simulink model "UnitTest_2"  (R2018b)
settings: Solver=FixedStepAuto  StartTime=0.0  StopTime=tfinal  FixedStep=1/30  RelTol=1e-3
values from neighbouring files (symbols this model uses):
  Bb = [14491; 3674; 39514] *1e-9    [UnitTestScript.m]
  Ri = [0.1;1;0.025]    [UnitTestScript.m]
libraries: aerolibutil x2, MEKF_lib x1
settings Model: Creator=kylle  LastModifiedBy=kylle

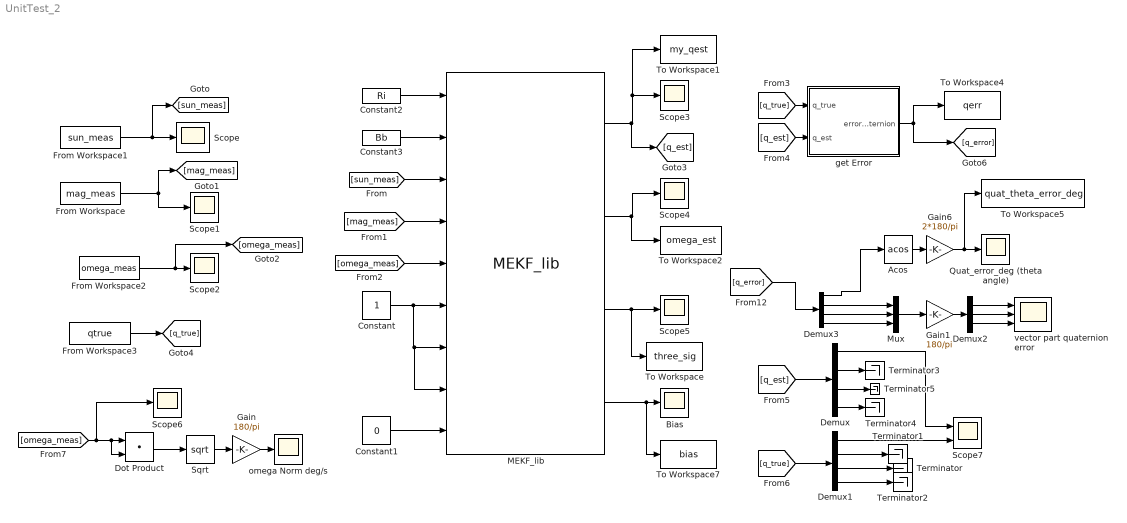
== system UnitTest_2 ==
  Acos : Trigonometry  Operator=acos
  Bias : Scope
  Constant : Constant
  Constant1 : Constant  Value=0
  Constant2 : Constant  Value=Ri
  Constant3 : Constant  Value=Bb
  Demux : Demux
  Demux1 : Demux
  Demux2 : Demux  Outputs=3
  Demux3 : Demux
  Dot Product : DotProduct  InputSameDT=on  OutDataTypeStr=Inherit: Inherit via internal rule
  From Workspace : FromWorkspace  VariableName=mag_meas  SampleTime=0
  From Workspace1 : FromWorkspace  VariableName=sun_meas  SampleTime=0
  From Workspace2 : FromWorkspace  VariableName=omega_meas  SampleTime=0
  From Workspace3 : FromWorkspace  VariableName=qtrue  SampleTime=0
  Gain : Gain  Gain=180/pi
  Gain1 : Gain  Gain=180/pi
  Gain6 : Gain  Gain=2*180/pi
  MEKF_lib : MEKF_lib/MEKF_lib  SystemSampleTime=-1
  Mux : Mux  Inputs=3
  Quat_error_deg (theta angle) : Scope
  Scope{,1..6} (7 alike) : Scope
  Scope7 : Scope  NumInputPorts=2
  Sqrt : Sqrt  SaturateOnIntegerOverflow=on
  Terminator{,1..5} (6 alike) : Terminator
  To Workspace : ToWorkspace  VariableName=three_sig  SaveFormat=Structure With Time  SampleTime=-1
  To Workspace1 : ToWorkspace  VariableName=my_qest  SaveFormat=Structure With Time  SampleTime=-1
  To Workspace2 : ToWorkspace  VariableName=omega_est  SaveFormat=Structure  SampleTime=-1
  To Workspace4 : ToWorkspace  VariableName=qerr  SaveFormat=Structure With Time  SampleTime=-1
  To Workspace5 : ToWorkspace  VariableName=quat_theta_error_deg  SaveFormat=Structure With Time  SampleTime=-1
  To Workspace7 : ToWorkspace  VariableName=bias  SaveFormat=Structure With Time  SampleTime=-1
  get Error : Subsystem
  omega Norm deg/s : Scope
  vector part quaternion error : Scope  NumInputPorts=3
  wires:
  Constant/1 -> MEKF_lib/8, MEKF_lib/7, MEKF_lib/6
  From Workspace1/1 -> [sun_meas], Scope/1
  From Workspace/1 -> [mag_meas], Scope1/1
  From Workspace2/1 -> [omega_meas], Scope2/1
  get Error/1(error_quaternion) -> To Workspace4/1, [q_error]
  [q_est] -> get Error/2(q_est)
  [q_true] -> get Error/1(q_true)
  From Workspace3/1 -> [q_true]
  Gain6/1 -> To Workspace5/1, Quat_error_deg (theta angle)/1
  Demux3/1 -> Acos/1
  Acos/1 -> Gain6/1
  [q_error] -> Demux3/1
  [q_est] -> Demux/1
  Demux/1 -> Scope7/1
  [q_true] -> Demux1/1
  Demux1/1 -> Scope7/2
  Demux1/3 -> Terminator/1
  Demux1/2 -> Terminator1/1
  Demux1/4 -> Terminator2/1
  Demux/2 -> Terminator3/1
  Demux/4 -> Terminator4/1
  Demux/3 -> Terminator5/1
  [omega_meas] -> Scope6/1, Dot Product/2, Dot Product/1
  Dot Product/1 -> Sqrt/1
  Sqrt/1 -> Gain/1
  Gain/1 -> omega Norm deg/s/1
  Demux3/2 -> Mux/1
  Demux3/3 -> Mux/2
  Demux3/4 -> Mux/3
  Mux/1 -> Gain1/1
  Gain1/1 -> Demux2/1
  Demux2/1 -> vector part quaternion error/1
  Demux2/2 -> vector part quaternion error/2
  Demux2/3 -> vector part quaternion error/3
  Constant2/1 -> MEKF_lib/1
  Constant3/1 -> MEKF_lib/2
  [sun_meas] -> MEKF_lib/3
  [mag_meas] -> MEKF_lib/4
  [omega_meas] -> MEKF_lib/5
  Constant1/1 -> MEKF_lib/9
  MEKF_lib/1 -> [q_est], Scope3/1, To Workspace1/1
  MEKF_lib/2 -> To Workspace2/1, Scope4/1
  MEKF_lib/3 -> To Workspace/1, Scope5/1
  MEKF_lib/4 -> To Workspace7/1, Bias/1

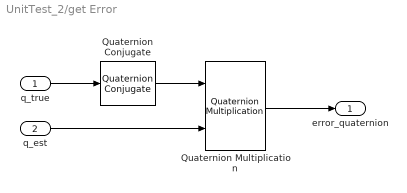
== system UnitTest_2/get Error ==
  q_true : Inport
  q_est : Inport  Port=2
  Quaternion Conjugate : aerolibutil/Quaternion Conjugate
      settings: SourceProductName=Aerospace Blockset  SourceProductBaseCode=AE
  Quaternion Multiplication : aerolibutil/Quaternion Multiplication
  error_quaternion : Outport
  wires:
  Quaternion Conjugate/1 -> Quaternion Multiplication/1
  Quaternion Multiplication/1 -> error_quaternion/1
  q_true/1 -> Quaternion Conjugate/1
  q_est/1 -> Quaternion Multiplication/2
